simulink model "FG_SIMU"  (R2021b)
settings: Solver=VariableStepAuto  StartTime=0.0  StopTime=10.0  RelTol=1e-3
values from neighbouring files (symbols this model uses):
  thetas_PD = [states_PD.theta]    [PD_SIM_CODE.m]    (also in PTS_SIM_CODE.m)
  y1s_PD = [statesdisp_PD.y1]    [PD_SIM_CODE.m]    (also in PTS_SIM_CODE.m)
  y2s_PD = [statesdisp_PD.y2]    [PD_SIM_CODE.m]    (also in PTS_SIM_CODE.m)
undefined symbols (not defined in the file or in its folder): Earth, WGS84
libraries: aerolibtransform2 x1, aerolibfltsims x1
settings Model: Creator=ccortes9  LastModifiedBy=ccortes9

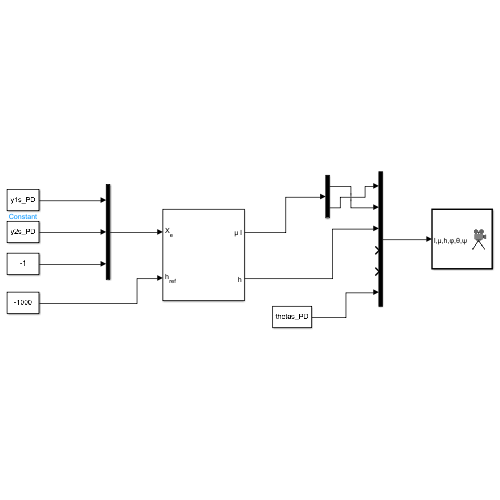
[thumbnail: Simulink's stored preview of the top-level diagram]
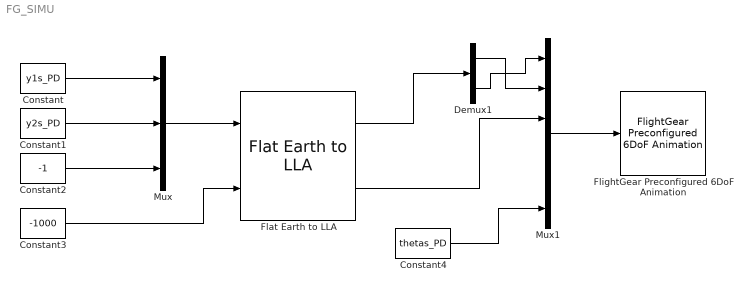
== system FG_SIMU ==
  Constant : Constant  Value=y1s_PD
  Constant1 : Constant  Value=y2s_PD
  Constant2 : Constant  Value=-1
  Constant3 : Constant  Value=-1000
  Constant4 : Constant  Value=thetas_PD
  Demux1 : Demux  Outputs=2
  Flat Earth to LLA : aerolibtransform2/Flat Earth to LLA  units=Metric (MKS)  ptype=Earth (WGS84)  F=1/298.257223563  R=6378137  refPosPort=off  LL0=[0 10]  psi=0
  FlightGear Preconfigured 6DoF Animation : aerolibfltsims/FlightGear Preconfigured 6DoF Animation  xFlightGearVersion=v2019.1  DestinationIpAddress=127.0.0.1  DestinationPort=5502  SampleTime=1/30  packetVersion=24
  Mux : Mux  Inputs=3
  Mux1 : Mux  Inputs=6
  wires:
  Mux/1 -> Flat Earth to LLA/1
  Constant/1 -> Mux/1
  Constant1/1 -> Mux/2
  Constant2/1 -> Mux/3
  Constant3/1 -> Flat Earth to LLA/2
  Mux1/1 -> FlightGear Preconfigured 6DoF Animation/1
  Flat Earth to LLA/1 -> Demux1/1
  Demux1/1 -> Mux1/2
  Demux1/2 -> Mux1/1
  Flat Earth to LLA/2 -> Mux1/3
  Constant4/1 -> Mux1/6
